simulink model "Project_Rocket"  (R2022a)
settings: Solver=VariableStepAuto  StartTime=0.0  StopTime=10.0  RelTol=1e-3
settings Model: Creator=LabPC  LastModifiedBy=LabPC

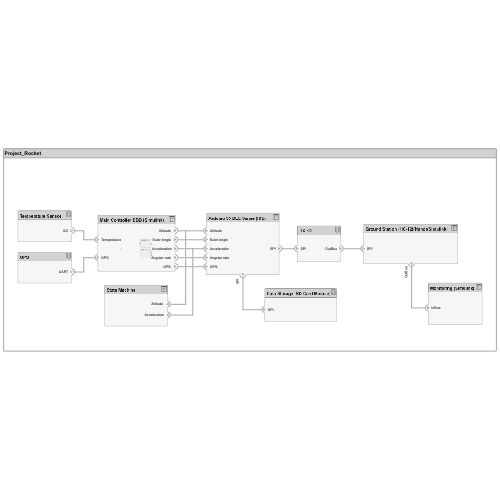
[thumbnail: Simulink's stored preview of the top-level diagram]
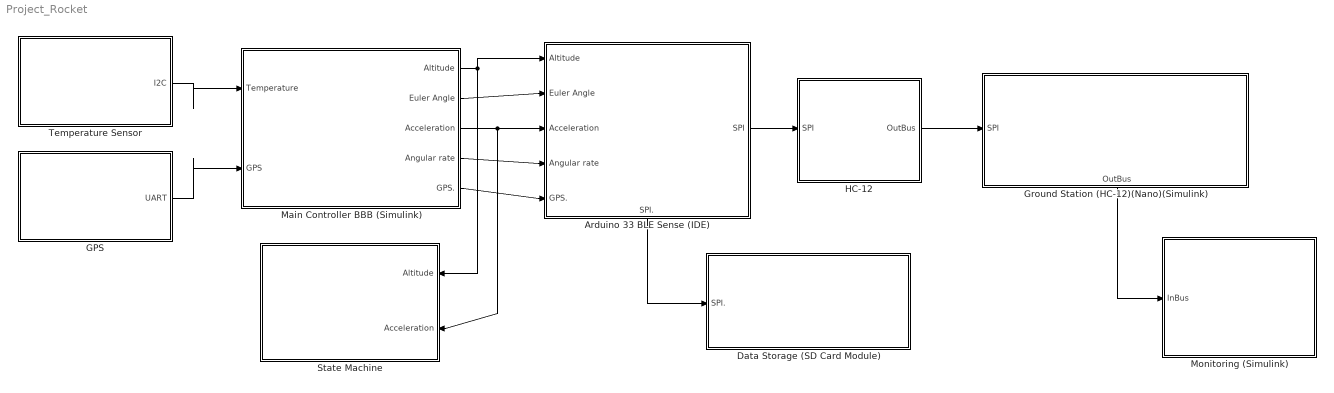
== system Project_Rocket ==
  Arduino 33 BLE Sense (IDE) : Subsystem
      settings: PortSchema="{\"entries\":[{\"content\":{\"headerSize\":26,\"margin\":15,\"minimumSpacing\":25,\"sides\":[{\"content\":{\"connectorIds\":[\"In1\",\"In2\",\"In3\",\"In4\",\"In5\"]},\"type\":\"ConnectorPlacement.EquallySpacedRectSide\",\"uuid\":\"979fab24-04cc-49c1-8140-29f72d9260c8\"},{\"content\":{\"connectorIds\":[\"Out2\"],\"side\":\"RIGHT\"},\"type\":\"ConnectorPlacement.EquallySpacedRectSide\",\"uuid\":\"0227c8ae-fbde-424f-bc98-340f6aa009e4\"},{\"content\":{\"connectorIds\":[],\"side\":\"TOP\"},\"type\":\"ConnectorPlacement.EquallySpacedRectSide\",\"uuid\":\"b75391ee-22da-429d-825c-2e8953c3d664\"},{\"content\":{\"connectorIds\":[\"Out1\"],\"side\":\"BOTTOM\"},\"type\":\"ConnectorPlacement.EquallySpacedRectSide\",\"uuid\":\"32757695-a988-44a2-9279-0809b7c97cfc\"}]},\"type\":\"ConnectorPlacement.EquallySpacedConnector\",\"uuid\":\"14a37765-6fcb-4736-a7a1-21d30d8061c8\"}],\"packageUris\":[\"http://schema.mathworks.com/mf0/Connector/R2020b\"],\"version\":\"1.0\"}"
  "Data Storage (SD Card Module) " : Subsystem
      settings: PortSchema="{\"entries\":[{\"content\":{\"headerSize\":26,\"margin\":15,\"minimumSpacing\":25,\"sides\":[{\"content\":{\"connectorIds\":[\"In1\"]},\"type\":\"ConnectorPlacement.EquallySpacedRectSide\",\"uuid\":\"979fab24-04cc-49c1-8140-29f72d9260c8\"},{\"content\":{\"connectorIds\":[],\"side\":\"RIGHT\"},\"type\":\"ConnectorPlacement.EquallySpacedRectSide\",\"uuid\":\"0227c8ae-fbde-424f-bc98-340f6aa009e4\"},{\"content\":{\"connectorIds\":[],\"side\":\"TOP\"},\"type\":\"ConnectorPlacement.EquallySpacedRectSide\",\"uuid\":\"b75391ee-22da-429d-825c-2e8953c3d664\"}]},\"type\":\"ConnectorPlacement.EquallySpacedConnector\",\"uuid\":\"14a37765-6fcb-4736-a7a1-21d30d8061c8\"}],\"packageUris\":[\"http://schema.mathworks.com/mf0/Connector/R2020b\"],\"version\":\"1.0\"}"
  "GPS " : Subsystem
      settings: PortSchema="{\"entries\":[{\"content\":{\"headerSize\":26,\"margin\":15,\"minimumSpacing\":25,\"sides\":[{\"content\":{\"connectorIds\":[]},\"type\":\"ConnectorPlacement.EquallySpacedRectSide\",\"uuid\":\"979fab24-04cc-49c1-8140-29f72d9260c8\"},{\"content\":{\"connectorIds\":[\"Out1\"],\"side\":\"RIGHT\"},\"type\":\"ConnectorPlacement.EquallySpacedRectSide\",\"uuid\":\"0227c8ae-fbde-424f-bc98-340f6aa009e4\"},{\"content\":{\"connectorIds\":[],\"side\":\"TOP\"},\"type\":\"ConnectorPlacement.EquallySpacedRectSide\",\"uuid\":\"b75391ee-22da-429d-825c-2e8953c3d664\"}]},\"type\":\"ConnectorPlacement.EquallySpacedConnector\",\"uuid\":\"14a37765-6fcb-4736-a7a1-21d30d8061c8\"}],\"packageUris\":[\"http://schema.mathworks.com/mf0/Connector/R2020b\"],\"version\":\"1.0\"}"
  "Ground Station (HC-12)(Nano)(Simulink) " : Subsystem
      settings: PortSchema="{\"entries\":[{\"content\":{\"headerSize\":26,\"margin\":15,\"minimumSpacing\":25,\"sides\":[{\"content\":{\"connectorIds\":[\"In1\"]},\"type\":\"ConnectorPlacement.EquallySpacedRectSide\",\"uuid\":\"979fab24-04cc-49c1-8140-29f72d9260c8\"},{\"content\":{\"connectorIds\":[],\"side\":\"RIGHT\"},\"type\":\"ConnectorPlacement.EquallySpacedRectSide\",\"uuid\":\"0227c8ae-fbde-424f-bc98-340f6aa009e4\"},{\"content\":{\"connectorIds\":[],\"side\":\"TOP\"},\"type\":\"ConnectorPlacement.EquallySpacedRectSide\",\"uuid\":\"b75391ee-22da-429d-825c-2e8953c3d664\"},{\"content\":{\"connectorIds\":[\"Out1\"],\"side\":\"BOTTOM\"},\"type\":\"ConnectorPlacement.EquallySpacedRectSide\",\"uuid\":\"b125680b-5c7d-4da5-92e2-1bb50a1e570a\"}]},\"type\":\"ConnectorPlacement.EquallySpacedConnector\",\"uuid\":\"14a37765-6fcb-4736-a7a1-21d30d8061c8\"}],\"packageUris\":[\"http://schema.mathworks.com/mf0/Connector/R2020b\"],\"version\":\"1.0\"}"
  HC-12 : Subsystem
      settings: PortSchema="{\"entries\":[{\"content\":{\"headerSize\":26,\"margin\":15,\"minimumSpacing\":25,\"sides\":[{\"content\":{\"connectorIds\":[\"In1\"]},\"type\":\"ConnectorPlacement.EquallySpacedRectSide\",\"uuid\":\"979fab24-04cc-49c1-8140-29f72d9260c8\"},{\"content\":{\"connectorIds\":[\"Out1\"],\"side\":\"RIGHT\"},\"type\":\"ConnectorPlacement.EquallySpacedRectSide\",\"uuid\":\"0227c8ae-fbde-424f-bc98-340f6aa009e4\"},{\"content\":{\"connectorIds\":[],\"side\":\"TOP\"},\"type\":\"ConnectorPlacement.EquallySpacedRectSide\",\"uuid\":\"b75391ee-22da-429d-825c-2e8953c3d664\"}]},\"type\":\"ConnectorPlacement.EquallySpacedConnector\",\"uuid\":\"14a37765-6fcb-4736-a7a1-21d30d8061c8\"}],\"packageUris\":[\"http://schema.mathworks.com/mf0/Connector/R2020b\"],\"version\":\"1.0\"}"
  "Main Controller BBB (Simulink) " : Subsystem
      settings: PortSchema="{\"entries\":[{\"content\":{\"headerSize\":26,\"margin\":15,\"minimumSpacing\":25,\"sides\":[{\"content\":{\"connectorIds\":[\"In1\",\"In2\"]},\"type\":\"ConnectorPlacement.EquallySpacedRectSide\",\"uuid\":\"979fab24-04cc-49c1-8140-29f72d9260c8\"},{\"content\":{\"connectorIds\":[\"Out1\",\"Out2\",\"Out3\",\"Out4\",\"Out5\"],\"side\":\"RIGHT\"},\"type\":\"ConnectorPlacement.EquallySpacedRectSide\",\"uuid\":\"0227c8ae-fbde-424f-bc98-340f6aa009e4\"},{\"content\":{\"connectorIds\":[],\"side\":\"TOP\"},\"type\":\"ConnectorPlacement.EquallySpacedRectSide\",\"uuid\":\"b75391ee-22da-429d-825c-2e8953c3d664\"}]},\"type\":\"ConnectorPlacement.EquallySpacedConnector\",\"uuid\":\"14a37765-6fcb-4736-a7a1-21d30d8061c8\"}],\"packageUris\":[\"http://schema.mathworks.com/mf0/Connector/R2020b\"],\"version\":\"1.0\"}"
  "Monitoring (Simulink) " : Subsystem
      settings: PortSchema="{\"entries\":[{\"content\":{\"headerSize\":26,\"margin\":15,\"minimumSpacing\":25,\"sides\":[{\"content\":{\"connectorIds\":[\"In1\"]},\"type\":\"ConnectorPlacement.EquallySpacedRectSide\",\"uuid\":\"979fab24-04cc-49c1-8140-29f72d9260c8\"},{\"content\":{\"connectorIds\":[],\"side\":\"RIGHT\"},\"type\":\"ConnectorPlacement.EquallySpacedRectSide\",\"uuid\":\"0227c8ae-fbde-424f-bc98-340f6aa009e4\"},{\"content\":{\"connectorIds\":[],\"side\":\"TOP\"},\"type\":\"ConnectorPlacement.EquallySpacedRectSide\",\"uuid\":\"b75391ee-22da-429d-825c-2e8953c3d664\"}]},\"type\":\"ConnectorPlacement.EquallySpacedConnector\",\"uuid\":\"14a37765-6fcb-4736-a7a1-21d30d8061c8\"}],\"packageUris\":[\"http://schema.mathworks.com/mf0/Connector/R2020b\"],\"version\":\"1.0\"}"
  "State Machine " : Subsystem
      settings: PortSchema="{\"entries\":[{\"content\":{\"headerSize\":26,\"margin\":15,\"minimumSpacing\":25,\"sides\":[{\"content\":{\"connectorIds\":[]},\"type\":\"ConnectorPlacement.EquallySpacedRectSide\",\"uuid\":\"979fab24-04cc-49c1-8140-29f72d9260c8\"},{\"content\":{\"connectorIds\":[\"In1\",\"In2\"],\"side\":\"RIGHT\"},\"type\":\"ConnectorPlacement.EquallySpacedRectSide\",\"uuid\":\"0227c8ae-fbde-424f-bc98-340f6aa009e4\"},{\"content\":{\"connectorIds\":[],\"side\":\"TOP\"},\"type\":\"ConnectorPlacement.EquallySpacedRectSide\",\"uuid\":\"b75391ee-22da-429d-825c-2e8953c3d664\"}]},\"type\":\"ConnectorPlacement.EquallySpacedConnector\",\"uuid\":\"14a37765-6fcb-4736-a7a1-21d30d8061c8\"}],\"packageUris\":[\"http://schema.mathworks.com/mf0/Connector/R2020b\"],\"version\":\"1.0\"}"
  "Temperature Sensor " : Subsystem
      settings: PortSchema="{\"entries\":[{\"content\":{\"headerSize\":26,\"margin\":15,\"minimumSpacing\":25,\"sides\":[{\"content\":{\"connectorIds\":[]},\"type\":\"ConnectorPlacement.EquallySpacedRectSide\",\"uuid\":\"979fab24-04cc-49c1-8140-29f72d9260c8\"},{\"content\":{\"connectorIds\":[\"Out1\"],\"side\":\"RIGHT\"},\"type\":\"ConnectorPlacement.EquallySpacedRectSide\",\"uuid\":\"0227c8ae-fbde-424f-bc98-340f6aa009e4\"},{\"content\":{\"connectorIds\":[],\"side\":\"TOP\"},\"type\":\"ConnectorPlacement.EquallySpacedRectSide\",\"uuid\":\"b75391ee-22da-429d-825c-2e8953c3d664\"}]},\"type\":\"ConnectorPlacement.EquallySpacedConnector\",\"uuid\":\"14a37765-6fcb-4736-a7a1-21d30d8061c8\"}],\"packageUris\":[\"http://schema.mathworks.com/mf0/Connector/R2020b\"],\"version\":\"1.0\"}"
  wires:
  "Temperature Sensor "/1(I2C) -> "Main Controller BBB (Simulink) "/1("Temperature ")
  "GPS "/1(UART) -> "Main Controller BBB (Simulink) "/2(GPS)
  "Main Controller BBB (Simulink) "/1("Altitude ") -> "State Machine "/1("Altitude "), Arduino 33 BLE Sense (IDE)/1("Altitude ")
  "Main Controller BBB (Simulink) "/2("Euler Angle ") -> Arduino 33 BLE Sense (IDE)/2("Euler Angle ")
  "Main Controller BBB (Simulink) "/3(Acceleration) -> "State Machine "/2(Acceleration), Arduino 33 BLE Sense (IDE)/3(Acceleration)
  "Main Controller BBB (Simulink) "/4("Angular rate ") -> Arduino 33 BLE Sense (IDE)/4("Angular rate ")
  "Main Controller BBB (Simulink) "/5(GPS.) -> Arduino 33 BLE Sense (IDE)/5(GPS.)
  Arduino 33 BLE Sense (IDE)/2(SPI) -> HC-12/1(SPI)
  HC-12/1(OutBus) -> "Ground Station (HC-12)(Nano)(Simulink) "/1(SPI)
  Arduino 33 BLE Sense (IDE)/1(SPI.) -> "Data Storage (SD Card Module) "/1(SPI.)
  "Ground Station (HC-12)(Nano)(Simulink) "/1(OutBus) -> "Monitoring (Simulink) "/1(InBus)

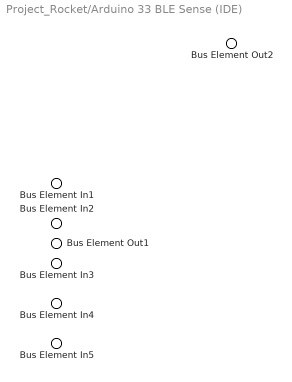
== system Project_Rocket/Arduino 33 BLE Sense (IDE) ==
  Bus Element In1 : Inport  PortName=Altitude
  Bus Element In2 : Inport  Port=2  PortName=Euler Angle
  Bus Element In3 : Inport  Port=3  PortName=Acceleration
  Bus Element In4 : Inport  Port=4  PortName=Angular rate
  Bus Element In5 : Inport  Port=5  PortName=GPS.
  Bus Element Out2 : Outport  PortName=SPI.
  Bus Element Out1 : Outport  Port=2  PortName=SPI

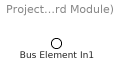
== system Project_Rocket/Data Storage (SD Card Module)  ==
  Bus Element In1 : Inport  PortName=SPI.

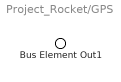
== system Project_Rocket/GPS  ==
  Bus Element Out1 : Outport  PortName=UART

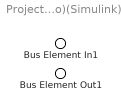
== system Project_Rocket/Ground Station (HC-12)(Nano)(Simulink)  ==
  Bus Element In1 : Inport  PortName=SPI
  Bus Element Out1 : Outport  PortName=OutBus

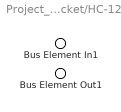
== system Project_Rocket/HC-12 ==
  Bus Element In1 : Inport  PortName=SPI
  Bus Element Out1 : Outport  PortName=OutBus

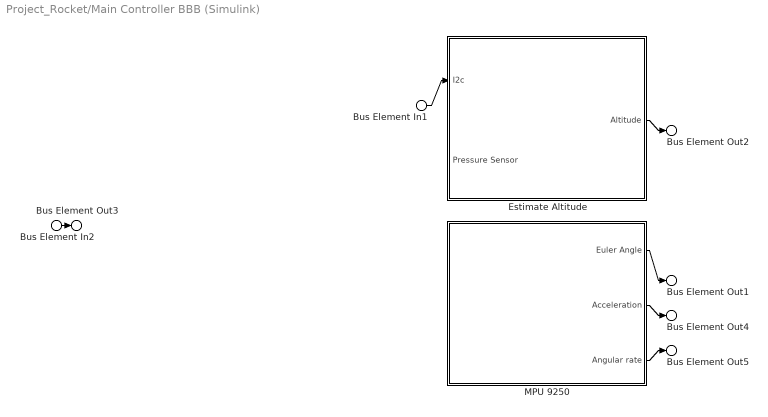
== system Project_Rocket/Main Controller BBB (Simulink)  ==
  Bus Element In1 : Inport  PortName=Temperature
  Bus Element In2 : Inport  Port=2  PortName=GPS
  "Estimate Altitude " : Subsystem
      settings: PortSchema="{\"entries\":[{\"content\":{\"headerSize\":26,\"margin\":15,\"minimumSpacing\":25,\"sides\":[{\"content\":{\"connectorIds\":[\"In1\",\"In2\"]},\"type\":\"ConnectorPlacement.EquallySpacedRectSide\",\"uuid\":\"979fab24-04cc-49c1-8140-29f72d9260c8\"},{\"content\":{\"connectorIds\":[\"Out1\"],\"side\":\"RIGHT\"},\"type\":\"ConnectorPlacement.EquallySpacedRectSide\",\"uuid\":\"0227c8ae-fbde-424f-bc98-340f6aa009e4\"},{\"content\":{\"connectorIds\":[],\"side\":\"TOP\"},\"type\":\"ConnectorPlacement.EquallySpacedRectSide\",\"uuid\":\"b75391ee-22da-429d-825c-2e8953c3d664\"}]},\"type\":\"ConnectorPlacement.EquallySpacedConnector\",\"uuid\":\"14a37765-6fcb-4736-a7a1-21d30d8061c8\"}],\"packageUris\":[\"http://schema.mathworks.com/mf0/Connector/R2020b\"],\"version\":\"1.0\"}"
  MPU 9250 : Subsystem
      settings: PortSchema="{\"entries\":[{\"content\":{\"headerSize\":26,\"margin\":15,\"minimumSpacing\":25,\"sides\":[{\"content\":{\"connectorIds\":[]},\"type\":\"ConnectorPlacement.EquallySpacedRectSide\",\"uuid\":\"979fab24-04cc-49c1-8140-29f72d9260c8\"},{\"content\":{\"connectorIds\":[\"Out1\",\"Out2\",\"Out3\"],\"side\":\"RIGHT\"},\"type\":\"ConnectorPlacement.EquallySpacedRectSide\",\"uuid\":\"0227c8ae-fbde-424f-bc98-340f6aa009e4\"},{\"content\":{\"connectorIds\":[],\"side\":\"TOP\"},\"type\":\"ConnectorPlacement.EquallySpacedRectSide\",\"uuid\":\"b75391ee-22da-429d-825c-2e8953c3d664\"}]},\"type\":\"ConnectorPlacement.EquallySpacedConnector\",\"uuid\":\"14a37765-6fcb-4736-a7a1-21d30d8061c8\"}],\"packageUris\":[\"http://schema.mathworks.com/mf0/Connector/R2020b\"],\"version\":\"1.0\"}"
  Bus Element Out2 : Outport  PortName=Altitude
  Bus Element Out1 : Outport  Port=2  PortName=Euler Angle
  Bus Element Out4 : Outport  Port=3  PortName=Acceleration
  Bus Element Out5 : Outport  Port=4  PortName=Angular rate
  Bus Element Out3 : Outport  Port=5  PortName=GPS.
  wires:
  Bus Element In1/1 -> "Estimate Altitude "/1(I2c)
  "Estimate Altitude "/1("Altitude ") -> Bus Element Out2/1
  Bus Element In2/1 -> Bus Element Out3/1
  MPU 9250/1("Euler Angle ") -> Bus Element Out1/1
  MPU 9250/2(Acceleration) -> Bus Element Out4/1
  MPU 9250/3("Angular rate ") -> Bus Element Out5/1

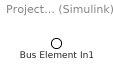
== system Project_Rocket/Monitoring (Simulink)  ==
  Bus Element In1 : Inport  PortName=InBus

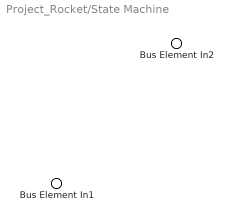
== system Project_Rocket/State Machine  ==
  Bus Element In2 : Inport  PortName=Altitude
  Bus Element In1 : Inport  Port=2  PortName=Acceleration

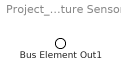
== system Project_Rocket/Temperature Sensor  ==
  Bus Element Out1 : Outport  PortName=I2C

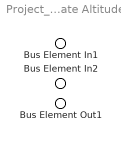
== system Project_Rocket/Main Controller BBB (Simulink) /Estimate Altitude  ==
  Bus Element In1 : Inport  PortName=I2c
  Bus Element In2 : Inport  Port=2  PortName=Pressure Sensor
  Bus Element Out1 : Outport  PortName=Altitude

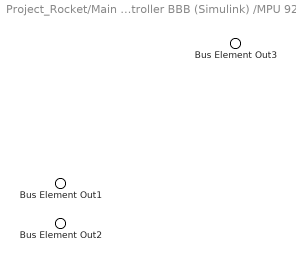
== system Project_Rocket/Main Controller BBB (Simulink) /MPU 9250 ==
  Bus Element Out1 : Outport  PortName=Euler Angle
  Bus Element Out3 : Outport  Port=2  PortName=Acceleration
  Bus Element Out2 : Outport  Port=3  PortName=Angular rate
